simulink model "Control_Arduino_SIM"  (R2023b)
settings: Solver=FixedStepAuto  StartTime=0.0  StopTime=90  RelTol=1e-3  EnableMultiTasking=on
undefined symbols (not defined in the file): L, R
libraries: arduinowifilib x2
settings Model: ExtModeTrigDuration=2  Creator=pablo  LastModifiedBy=pablo
settings OptimizationCC: EnhancedBackFolding=on  PassReuseOutputArgsAs=Individual arguments  ZeroExternalMemoryAtStartup=off  ZeroInternalMemoryAtStartup=off  MaxStackSize=64  OptimizeBlockOrder=speed  DifferentSizesBufferReuse=on  OptimizationCustomize=off  EfficientTunableParamExpr=on
settings DebuggingCC: ParameterTunabilityLossMsg=error
settings HardwareCC: ProdBitPerPointer=32  ProdBitPerSizeT=32  ProdBitPerPtrDiffT=32  ProdLargestAtomicInteger=Long  ProdLargestAtomicFloat=Double  ProdWordSize=32  ProdHWDeviceType=ARM Compatible->ARM Cortex
settings SFSimCC: MATLABDynamicMemAlloc=off
settings RTWCC: Description=Embedded Coder  SystemTargetFile=ert.tlc  HardwareBoard=Arduino MKR WiFi 1010  TemplateMakefile=ert_default_tmf  Toolchain=Arduino ARM  BuildConfiguration=Faster Runs
settings CodeAppCC: ForceParamTrailComments=on  IgnoreCustomStorageClasses=off  OperatorAnnotations=on  SimulinkDataObjDesc=on  SFDataObjDesc=on  InsertBlockDesc=on
settings ERTTargetCC: SupportContinuousTime=on  SupportVariableSizeSignals=on  ExtModeTransport=3  ExtModeStaticAlloc=on  ExtModeAutomaticAllocSize=off  ExtModeStaticAllocSize=8192  ExtModeMexFile=ext_xcp  ExtModeIntrfLevel=Level2 - Open

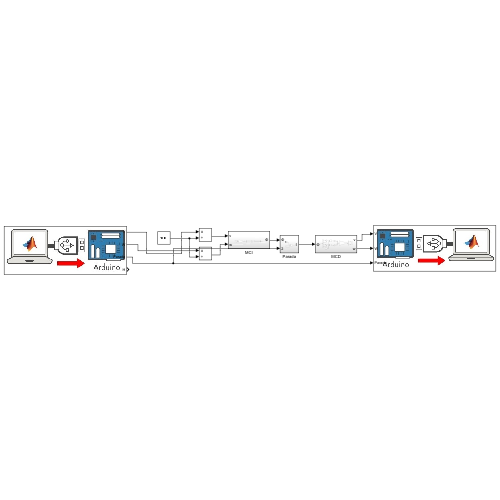
[thumbnail: Simulink's stored preview of the top-level diagram]
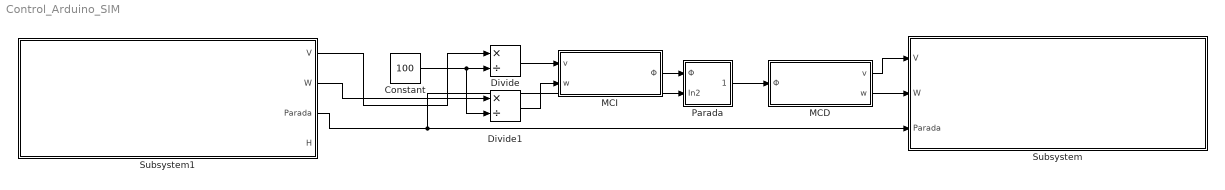
== system Control_Arduino_SIM ==
  Constant : Constant  Value=100
  Divide : Product  Inputs=*/
  Divide1 : Product  Inputs=*/
  MCD : Subsystem
  MCI : Subsystem
  Parada : Subsystem
  Subsystem : Subsystem
      mask Display: image('am.jpg');
  Subsystem1 : Subsystem
      mask Display: image('ma.jpg');
  wires:
  Constant/1 -> Divide1/2, Divide/2
  Parada/1(Out1) -> MCD/1(Φ)
  MCI/1(Φ) -> Parada/1(Φ)
  Subsystem1/1(V) -> Divide/1
  Subsystem1/2(W) -> Divide1/1
  Subsystem1/3(Parada) -> Subsystem/3(Parada), Parada/2(In2)
  Divide1/1 -> MCI/2(w)
  Divide/1 -> MCI/1(v)
  MCD/1(v) -> Subsystem/1(V)
  MCD/2(w) -> Subsystem/2(W)

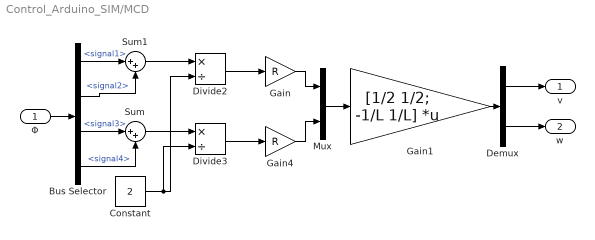
== system Control_Arduino_SIM/MCD ==
  Φ : Inport
  Bus Selector : BusSelector  OutputSignals=signal1,signal2,signal3,signal4
  Constant : Constant  Value=2
  Demux : Demux  Outputs=2
  Divide2 : Product  Inputs=*/
  Divide3 : Product  Inputs=*/
  Gain : Gain  Gain=R
  Gain1 : Gain  Gain=[1/2 1/2; -1/L 1/L]  Multiplication=Matrix(K*u) (u vector)
  Gain4 : Gain  Gain=R
  Mux : Mux  Inputs=2
  Sum : Sum  Inputs=|++
  Sum1 : Sum  Inputs=|++
  v : Outport
  w : Outport  Port=2
  wires:
  Sum1/1 -> Divide2/1
  Bus Selector/1 -> Sum1/1  "<signal1>"
  Φ/1 -> Bus Selector/1
  Divide2/1 -> Gain/1
  Bus Selector/4 -> Sum/2  "<signal4>"
  Bus Selector/3 -> Sum/1  "<signal3>"
  Bus Selector/2 -> Sum1/2  "<signal2>"
  Constant/1 -> Divide2/2, Divide3/2
  Sum/1 -> Divide3/1
  Divide3/1 -> Gain4/1
  Gain/1 -> Mux/1
  Gain4/1 -> Mux/2
  Mux/1 -> Gain1/1
  Gain1/1 -> Demux/1
  Demux/1 -> v/1
  Demux/2 -> w/1

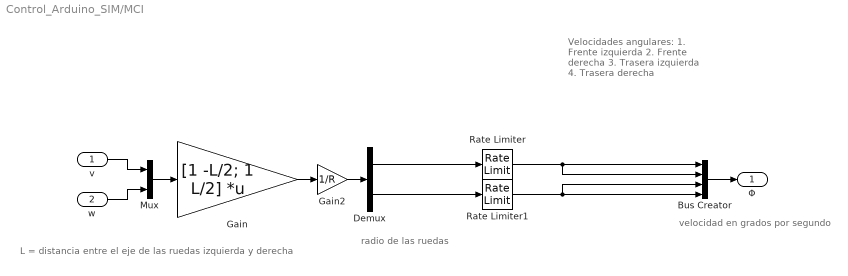
== system Control_Arduino_SIM/MCI ==
  note: velocidad en grados por segundo
  note: L = distancia entre el eje de las ruedas izquierda y derecha
  note: radio de las ruedas
  note: Velocidades angulares:
      | 1. Frente izquierda
      | 2. Frente derecha
      | 3. Trasera izquierda
      | 4. Trasera derecha
  v : Inport
  w : Inport  Port=2
  Bus Creator : BusCreator  Inputs=4
  Demux : Demux  Outputs=2
  Gain : Gain  Gain=[1 -L/2; 1 L/2]  Multiplication=Matrix(K*u) (u vector)
  Gain2 : Gain  Gain=1/R
  Mux : Mux  Inputs=2
  Rate Limiter : RateLimiter  RisingSlewLimit=9  FallingSlewLimit=-9  SampleTimeMode=inherited
  Rate Limiter1 : RateLimiter  RisingSlewLimit=9  FallingSlewLimit=-9  SampleTimeMode=inherited
  Φ : Outport
  wires:
  Bus Creator/1 -> Φ/1
  Mux/1 -> Gain/1
  v/1 -> Mux/1
  w/1 -> Mux/2
  Demux/1 -> Rate Limiter/1
  Demux/2 -> Rate Limiter1/1
  Gain/1 -> Gain2/1
  Gain2/1 -> Demux/1
  Rate Limiter/1 -> Bus Creator/2, Bus Creator/1
  Rate Limiter1/1 -> Bus Creator/4, Bus Creator/3

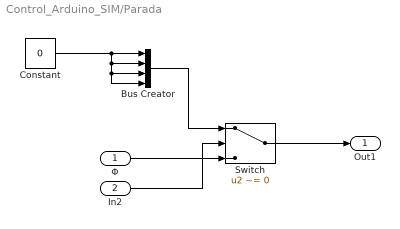
== system Control_Arduino_SIM/Parada ==
  Φ : Inport
  In2 : Inport  Port=2
  Bus Creator : BusCreator  Inputs=4
  Constant : Constant  Value=0
  Switch : Switch  Criteria=u2 ~= 0  SaturateOnIntegerOverflow=off  InputSameDT=off
  Out1 : Outport
  wires:
  Switch/1 -> Out1/1
  Φ/1 -> Switch/3
  In2/1 -> Switch/2
  Bus Creator/1 -> Switch/1
  Constant/1 -> Bus Creator/4, Bus Creator/3, Bus Creator/2, Bus Creator/1

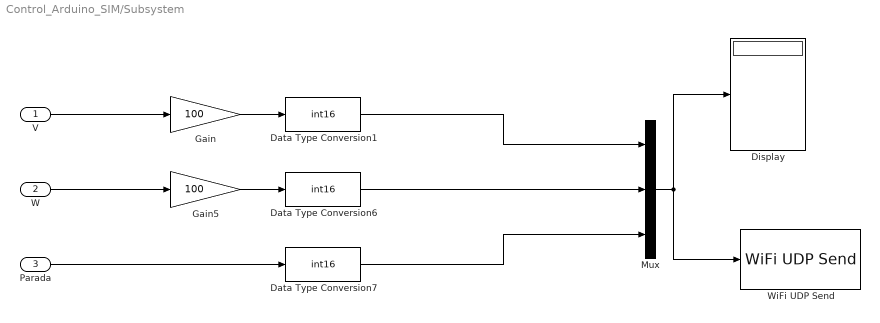
== system Control_Arduino_SIM/Subsystem ==
  V : Inport
  W : Inport  Port=2
  Parada : Inport  Port=3
  Data Type Conversion1 : DataTypeConversion  OutDataTypeStr=int16  ConvertRealWorld=Stored Integer (SI)  SaturateOnIntegerOverflow=off  RndMeth=Floor
  Data Type Conversion6 : DataTypeConversion  OutDataTypeStr=int16  ConvertRealWorld=Stored Integer (SI)  SaturateOnIntegerOverflow=off  RndMeth=Floor
  Data Type Conversion7 : DataTypeConversion  OutDataTypeStr=int16  ConvertRealWorld=Stored Integer (SI)  SaturateOnIntegerOverflow=off  RndMeth=Floor
  Display : Display
  Gain : Gain  Gain=100
  Gain5 : Gain  Gain=100
  Mux : Mux  Inputs=3
  WiFi UDP Send : arduinowifilib/WiFi UDP Send  remoteIPOctetString=192.168.137.1  remoteport=8888  localport=9090  remoteipoctet1=192  remoteipoctet2=168  remoteipoctet3=137  remoteipoctet4=1  wifiUDPIndex=0  blockPlatform=ARDUINO  isARMArch=true
  wires:
  Mux/1 -> Display/1, WiFi UDP Send/1
  V/1 -> Gain/1
  W/1 -> Gain5/1
  Data Type Conversion6/1 -> Mux/2
  Data Type Conversion7/1 -> Mux/3
  Gain/1 -> Data Type Conversion1/1
  Gain5/1 -> Data Type Conversion6/1
  Parada/1 -> Data Type Conversion7/1
  Data Type Conversion1/1 -> Mux/1

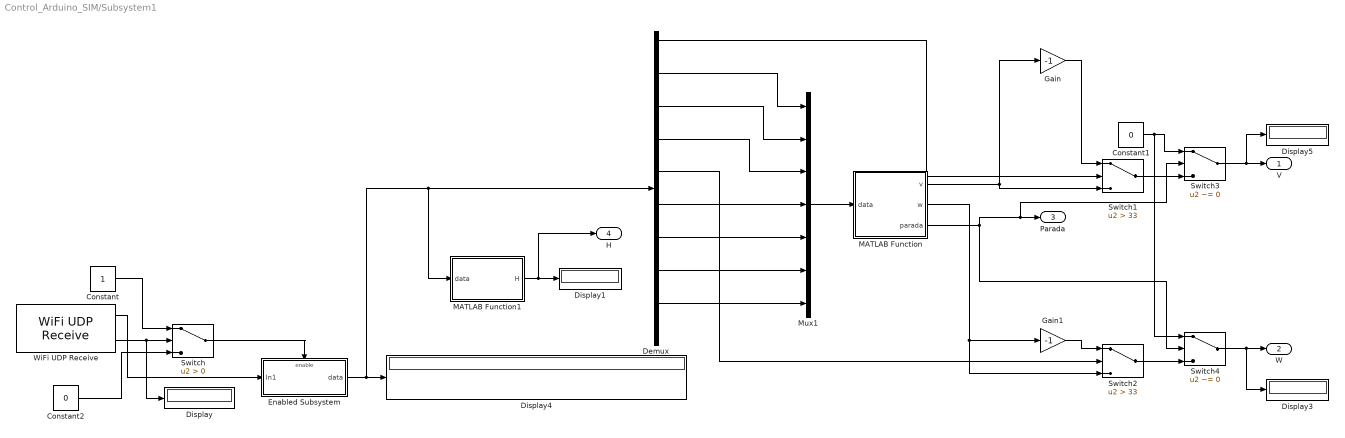
== system Control_Arduino_SIM/Subsystem1 ==
  Constant : Constant  OutDataTypeStr=boolean
  Constant1 : Constant  Value=0
  Constant2 : Constant  Value=0  OutDataTypeStr=boolean
  Demux : Demux  Outputs=10
  Display{,1,3..5} (5 alike) : Display
      Display1 settings: Format=binary (Stored Integer)
  Enabled Subsystem : Subsystem  TreatAsAtomicUnit=on
  Gain : Gain  Gain=-1
  Gain1 : Gain  Gain=-1
  MATLAB Function : MATLAB Function  TreatAsAtomicUnit=on
  MATLAB Function1 : MATLAB Function  TreatAsAtomicUnit=on
  Mux1 : Mux  Inputs=7
  Switch : Switch  Criteria=u2 > Threshold  SaturateOnIntegerOverflow=off  InputSameDT=off
  Switch1 : Switch  Criteria=u2 > Threshold  Threshold=33  SaturateOnIntegerOverflow=off  InputSameDT=off
  Switch2 : Switch  Criteria=u2 > Threshold  Threshold=33  SaturateOnIntegerOverflow=off  InputSameDT=off
  Switch3 : Switch  Criteria=u2 ~= 0  SaturateOnIntegerOverflow=off  InputSameDT=off
  Switch4 : Switch  Criteria=u2 ~= 0  SaturateOnIntegerOverflow=off  InputSameDT=off
  WiFi UDP Receive : arduinowifilib/WiFi UDP Receive  localport=9090  DataType=uint8  DataLength=10  SampleTime_=0.1  wifiUDPIndex=0  blockPlatform=ARDUINO  isARMArch=true
  V : Outport
  W : Outport  Port=2
  Parada : Outport  Port=3
  H : Outport  Port=4
  wires:
  Enabled Subsystem/1(data) -> Display4/1, Demux/1, MATLAB Function1/1(data)
  Constant/1 -> Switch/1
  WiFi UDP Receive/1 -> Enabled Subsystem/1(In1)
  Demux/1 -> Switch1/2
  Demux/2 -> Mux1/1
  WiFi UDP Receive/2 -> Switch/2, Display/1
  Demux/4 -> Mux1/3
  Demux/3 -> Mux1/2
  Switch/1 -> Enabled Subsystem/Enable
  Demux/6 -> Mux1/4
  Demux/5 -> Switch2/2
  Demux/8 -> Mux1/6
  Demux/7 -> Mux1/5
  Demux/9 -> Mux1/7
  Mux1/1 -> MATLAB Function/1(data)
  MATLAB Function/1(v) -> Switch1/3, Gain/1
  MATLAB Function/2(w) -> Switch2/3, Gain1/1
  MATLAB Function/3(parada) -> Switch4/2, Switch3/2, Parada/1
  Gain/1 -> Switch1/1
  Gain1/1 -> Switch2/1
  Constant1/1 -> Switch4/1, Switch3/1
  Switch2/1 -> Switch4/3
  Switch1/1 -> Switch3/3
  Switch4/1 -> W/1, Display3/1
  Switch3/1 -> V/1, Display5/1
  MATLAB Function1/1(H) -> H/1, Display1/1
  Constant2/1 -> Switch/3

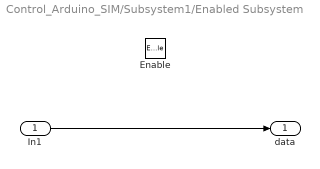
== system Control_Arduino_SIM/Subsystem1/Enabled Subsystem ==
  In1 : Inport
  Enable : EnablePort
  data : Outport
  wires:
  In1/1 -> data/1

== matlab function Control_Arduino_SIM/Subsystem1/MATLAB Function ==
  data: data input; v output; w output; parada output
function [v,w,parada] = data2vwparada(data)
parada=uint8(0);
v=single(0);
w=single(0);
d1=single(data(1)-48);
d2=single(data(2)-48);
d3=single(data(3)-48);
d4=single(data(4)-48);
d5=single(data(5)-48);
d6=single(data(6)-48);


v=single(d1*16^2+d2*16+d3);
w=single(d4*16^2+d5*16+d6);
parada=data(7)-48;

== matlab function Control_Arduino_SIM/Subsystem1/MATLAB Function1 ==
  data: data input; H output
function H  = extraerH(data)
H=data(10);
end
